simulink model "eg2"  (R2020a)
settings: Solver=VariableStepAuto  StartTime=0.0  StopTime=10.0  RelTol=1e-3
settings Model: Creator=DELL  LastModifiedBy=DELL

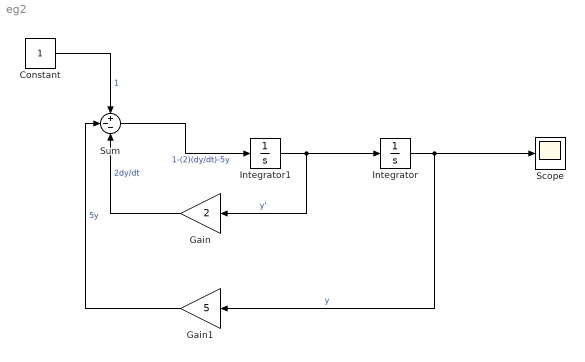
== system eg2 ==
  Constant : Constant
  Gain : Gain  Gain=2
  Gain1 : Gain  Gain=5
  Integrator : Integrator
  Integrator1 : Integrator
  Scope : Scope
  Sum : Sum  Inputs=+--
  wires:
  Integrator1/1 -> Gain/1, Integrator/1  "y'"
  Integrator/1 -> Scope/1, Gain1/1  "y"
  Constant/1 -> Sum/1  "1"
  Gain/1 -> Sum/3  "2dy/dt"
  Gain1/1 -> Sum/2  "5y"
  Sum/1 -> Integrator1/1  "1-(2)(dy/dt)-5y"
